simulink model "platoon_greedy_best_first_search"  (R2020b)
settings: Solver=VariableStepAuto  StartTime=0.0  StopTime=25.0  RelTol=1e-3
values from neighbouring files (symbols this model uses):
  loc = zeros(size)    [time_comparison.m]
undefined symbols (not defined in the file or in its folder): objects
libraries: mobileRoboticsLib x13, pid_lib x8
settings Model: Creator=Roozbeh  LastModifiedBy=Roozbeh

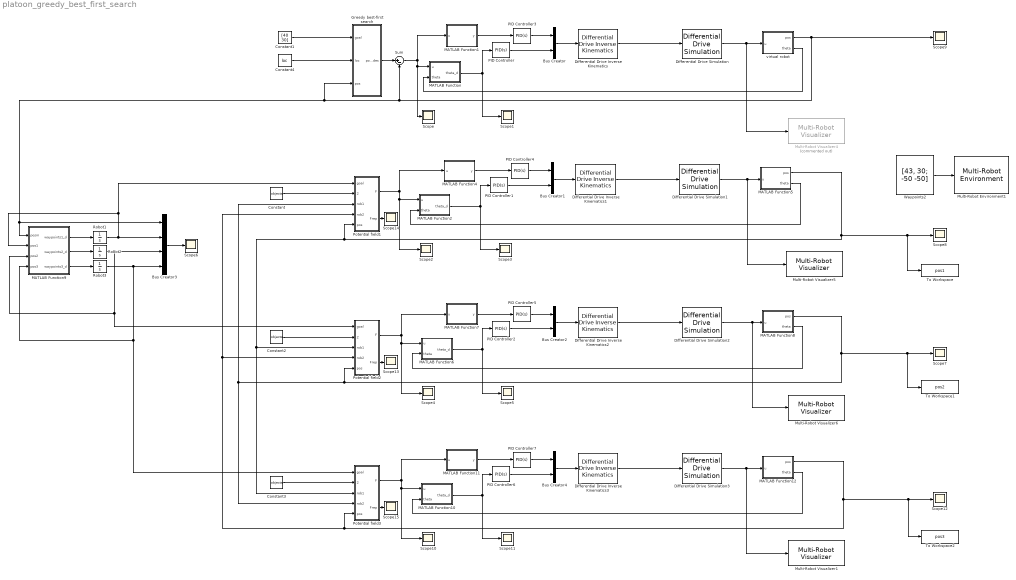
== system platoon_greedy_best_first_search ==
  Bus Creator{,1..2,4} (4 alike) : BusCreator  Inputs=2
  Bus Creator3 : BusCreator  Inputs=4
  Constant : Constant  Value=objects
  Constant1 : Constant  Value=[40 30]
  Constant2 : Constant  Value=objects
  Constant3 : Constant  Value=objects
  Constant4 : Constant  Value=loc
  Differential Drive Inverse Kinematics{,1..3} (4 alike) : mobileRoboticsLib/Kinematic Models/Differential Drive/Differential Drive Inverse Kinematics  wheelRadius=0.1  wheelBase=0.5
      settings: SourceProductName=Mobile Robotics Simulation Toolbox
  Differential Drive Simulation : mobileRoboticsLib/Kinematic Models/Differential Drive/Differential Drive Simulation  wheelRadius=0.1  wheelBase=0.5  initX=6  initY=6  initAngle=0  Ts=0.05
      settings: SourceProductName=Mobile Robotics Simulation Toolbox
  Differential Drive Simulation1 : mobileRoboticsLib/Kinematic Models/Differential Drive/Differential Drive Simulation  wheelRadius=0.1  wheelBase=0.5  initX=8  initY=8  initAngle=0  Ts=0.05
      settings: SourceProductName=Mobile Robotics Simulation Toolbox
  Differential Drive Simulation2 : mobileRoboticsLib/Kinematic Models/Differential Drive/Differential Drive Simulation  wheelRadius=0.1  wheelBase=0.5  initX=4  initY=4  initAngle=0  Ts=0.05
      settings: SourceProductName=Mobile Robotics Simulation Toolbox
  Differential Drive Simulation3 : mobileRoboticsLib/Kinematic Models/Differential Drive/Differential Drive Simulation  wheelRadius=0.1  wheelBase=0.5  initX=4  initY=12  initAngle=0  Ts=0.05
      settings: SourceProductName=Mobile Robotics Simulation Toolbox
  Greedy best-first search : MATLAB Function  TreatAsAtomicUnit=on
  MATLAB Function : MATLAB Function  TreatAsAtomicUnit=on
  MATLAB Function1 : MATLAB Function  TreatAsAtomicUnit=on
  MATLAB Function10 : MATLAB Function  TreatAsAtomicUnit=on
  MATLAB Function11 : MATLAB Function  TreatAsAtomicUnit=on
  MATLAB Function12 : MATLAB Function  TreatAsAtomicUnit=on
  MATLAB Function2 : MATLAB Function  TreatAsAtomicUnit=on
  MATLAB Function4 : MATLAB Function  TreatAsAtomicUnit=on
  MATLAB Function5 : MATLAB Function  TreatAsAtomicUnit=on
  MATLAB Function6 : MATLAB Function  TreatAsAtomicUnit=on
  MATLAB Function7 : MATLAB Function  TreatAsAtomicUnit=on
  MATLAB Function8 : MATLAB Function  TreatAsAtomicUnit=on
  MATLAB Function9 : MATLAB Function  TreatAsAtomicUnit=on
  Multi-Robot Environment1 : mobileRoboticsLib/Environments/Multi-Robot Environment  numRobots=3  mapName=mapRooz  showWaypoints=on  showObjects=off  objectColors=[ 1, 0, 0; 0, 1, 0; 0, 0, 1 ]  objectMarkers='s'  showRobotIds=on  plotSensorLines=on
      settings: SourceProductName=Mobile Robotics Simulation Toolbox
  Multi-Robot Visualizer1 : mobileRoboticsLib/Environments/Multi-Robot Visualizer  idx=3  radius=0.5  robotColor=[0 0 1]  showTraj=off  hasLidar=off  sensorOffset=[0,0]  scanAngles=[-pi/4 0 pi/4]  maxNumScans=0  hasObjDetector=off  objDetectorOffset=[0,0]  objDetectorAngle=0  objDetectorFOV=pi/3  objDetectorMaxRange=5  hasRobotDetector=off  robotDetectorOffset=[0,0]  robotDetectorAngle=0  robotDetectorFOV=pi/3  robotDetectorMaxRange=5  robotDetectorNumDetections=0
      settings: SourceProductName=Mobile Robotics Simulation Toolbox
  Multi-Robot Visualizer4 : mobileRoboticsLib/Environments/Multi-Robot Visualizer  Commented=on  idx=1  radius=0.5  robotColor=[0 0 1]  showTraj=off  hasLidar=off  sensorOffset=[0,0]  scanAngles=[-pi/4 0 pi/4]  maxNumScans=0  hasObjDetector=off  objDetectorOffset=[0,0]  objDetectorAngle=0  objDetectorFOV=pi/3  objDetectorMaxRange=5  hasRobotDetector=off  robotDetectorOffset=[0,0]  robotDetectorAngle=0  robotDetectorFOV=pi/3  robotDetectorMaxRange=5  robotDetectorNumDetections=0
      settings: SourceProductName=Mobile Robotics Simulation Toolbox
  Multi-Robot Visualizer5 : mobileRoboticsLib/Environments/Multi-Robot Visualizer  idx=1  radius=0.5  robotColor=[0 1 0]  showTraj=off  hasLidar=off  sensorOffset=[0,0]  scanAngles=[-pi/4 0 pi/4]  maxNumScans=0  hasObjDetector=off  objDetectorOffset=[0,0]  objDetectorAngle=0  objDetectorFOV=pi/3  objDetectorMaxRange=5  hasRobotDetector=off  robotDetectorOffset=[0,0]  robotDetectorAngle=0  robotDetectorFOV=pi/3  robotDetectorMaxRange=5  robotDetectorNumDetections=0
      settings: SourceProductName=Mobile Robotics Simulation Toolbox
  Multi-Robot Visualizer6 : mobileRoboticsLib/Environments/Multi-Robot Visualizer  idx=2  radius=0.5  robotColor=[1 0 0]  showTraj=off  hasLidar=off  sensorOffset=[0,0]  scanAngles=[-pi/4 0 pi/4]  maxNumScans=0  hasObjDetector=off  objDetectorOffset=[0,0]  objDetectorAngle=0  objDetectorFOV=pi/3  objDetectorMaxRange=5  hasRobotDetector=off  robotDetectorOffset=[0,0]  robotDetectorAngle=0  robotDetectorFOV=pi/3  robotDetectorMaxRange=5  robotDetectorNumDetections=0
      settings: SourceProductName=Mobile Robotics Simulation Toolbox
  PID Controller{,1..2,6} (4 alike) : pid_lib/PID Controller  Controller=PID  Form=Parallel  TimeDomain=Continuous-time  UseExternalTs=off  SampleTime=-1  IntegratorMethod=Forward Euler  FilterMethod=Forward Euler  ControllerParametersSource=internal  P=10  I=1  D=0  UseFilter=on  N=100  TunerSelectOption=Transfer Function Based (PID Tuner App)  InitialConditionSource=internal  InitialConditionForIntegrator=0  InitialConditionForFilter=0  DifferentiatorICPrevScaledInput=0  ExternalReset=none  TrackingMode=off  Kt=1  LimitOutput=off  SatLimitsSource=internal  UpperSaturationLimit=3  LowerSaturationLimit=-3  LinearizeAsGain=on  AntiWindupMode=none  Kb=1  POutMin=[]  POutMax=[]  IOutMin=[]  IOutMax=[]  DOutMin=[]  DOutMax=[]  NOutMin=[]  NOutMax=[]  SumOutMin=[]  SumOutMax=[]  SaturationOutMin=[]  SaturationOutMax=[]  PParamMin=[]  PParamMax=[]  IParamMin=[]  IParamMax=[]  DParamMin=[]  DParamMax=[]  NParamMin=[]  NParamMax=[]  KbParamMin=[]  KbParamMax=[]  KtParamMin=[]  KtParamMax=[]  KbOutMin=[]  KbOutMax=[]  KtOutMin=[]  KtOutMax=[]  IntegratorOutMin=[]  IntegratorOutMax=[]  FilterOutMin=[]  FilterOutMax=[]  SumI1OutMin=[]  SumI1OutMax=[]  SumI2OutMin=[]  SumI2OutMax=[]  SumI3OutMin=[]  SumI3OutMax=[]  SumI4OutMin=[]  SumI4OutMax=[]  SumDOutMin=[]  SumDOutMax=[]  DifferentiatorOutMin=[]  DifferentiatorOutMax=[]  FilterDiffOutCoefMin=[]  FilterDiffOutCoefMax=[]  ReciprocalOutMin=[]  ReciprocalOutMax=[]  SumDenOutMin=[]  SumDenOutMax=[]  SumNumOutMin=[]  SumNumOutMax=[]  DivideOutMin=[]  DivideOutMax=[]  UdiffTsProdOutMin=[]  UdiffTsProdOutMax=[]  NTsProdOutMin=[]  NTsProdOutMax=[]  UintegralTsProdOutMin=[]  UintegralTsProdOutMax=[]  UngainTsProdOutMin=[]  UngainTsProdOutMax=[]  IntegratorContinuousStateAttributes=''  IntegratorStateMustResolveToSignalObject=off  IntegratorRTWStateStorageClass=Auto  FilterContinuousStateAttributes=''  FilterStateMustResolveToSignalObject=off  FilterRTWStateStorageClass=Auto  ParallelPVariant=InternalParameters  IdealPVariant=Disabled  IVariant=InternalParameters  DVariant=InternalParameters  IntegratorVariant=Continuous  SatVariant=Disabled  AWVariant=Passthrough  PCopyVariant=Disabled  TRVariant=Disabled  FdbkBlocksVariant=Forward  IdealPFdbkVariant=Disabled  SatFdbkVariant=Disabled  DerivativeFilterVariant=ContFilter  NVariant=InternalParameters  NCopyVariant=Disabled  FilterICVariant=InternalICsFilter  IntegratorICVariant=InternalICs  ExternalResetVariant=Disabled  TRSumVariant=Passthrough  SumFdbkVariant=Disabled  SumVariant=Sum_PID  TsampFilterVariant=InternalTs  TsampNgainVariant=Passthrough  TsampIntegralVariant=Passthrough  ExternalSaturationOutDataTypeStr=Inherit: Same as second input
  PID Controller3 : pid_lib/PID Controller  Controller=PID  Form=Parallel  TimeDomain=Continuous-time  UseExternalTs=off  SampleTime=-1  IntegratorMethod=Forward Euler  FilterMethod=Forward Euler  ControllerParametersSource=internal  P=5  I=0  D=0.1  UseFilter=on  N=100  TunerSelectOption=Transfer Function Based (PID Tuner App)  InitialConditionSource=internal  InitialConditionForIntegrator=0  InitialConditionForFilter=0  DifferentiatorICPrevScaledInput=0  ExternalReset=none  TrackingMode=off  Kt=1  LimitOutput=on  SatLimitsSource=internal  UpperSaturationLimit=3  LowerSaturationLimit=-3  LinearizeAsGain=on  AntiWindupMode=none  Kb=1  POutMin=[]  POutMax=[]  IOutMin=[]  IOutMax=[]  DOutMin=[]  DOutMax=[]  NOutMin=[]  NOutMax=[]  SumOutMin=[]  SumOutMax=[]  SaturationOutMin=[]  SaturationOutMax=[]  PParamMin=[]  PParamMax=[]  IParamMin=[]  IParamMax=[]  DParamMin=[]  DParamMax=[]  NParamMin=[]  NParamMax=[]  KbParamMin=[]  KbParamMax=[]  KtParamMin=[]  KtParamMax=[]  KbOutMin=[]  KbOutMax=[]  KtOutMin=[]  KtOutMax=[]  IntegratorOutMin=[]  IntegratorOutMax=[]  FilterOutMin=[]  FilterOutMax=[]  SumI1OutMin=[]  SumI1OutMax=[]  SumI2OutMin=[]  SumI2OutMax=[]  SumI3OutMin=[]  SumI3OutMax=[]  SumI4OutMin=[]  SumI4OutMax=[]  SumDOutMin=[]  SumDOutMax=[]  DifferentiatorOutMin=[]  DifferentiatorOutMax=[]  FilterDiffOutCoefMin=[]  FilterDiffOutCoefMax=[]  ReciprocalOutMin=[]  ReciprocalOutMax=[]  SumDenOutMin=[]  SumDenOutMax=[]  SumNumOutMin=[]  SumNumOutMax=[]  DivideOutMin=[]  DivideOutMax=[]  UdiffTsProdOutMin=[]  UdiffTsProdOutMax=[]  NTsProdOutMin=[]  NTsProdOutMax=[]  UintegralTsProdOutMin=[]  UintegralTsProdOutMax=[]  UngainTsProdOutMin=[]  UngainTsProdOutMax=[]  IntegratorContinuousStateAttributes=''  IntegratorStateMustResolveToSignalObject=off  IntegratorRTWStateStorageClass=Auto  FilterContinuousStateAttributes=''  FilterStateMustResolveToSignalObject=off  FilterRTWStateStorageClass=Auto  ParallelPVariant=InternalParameters  IdealPVariant=Disabled  IVariant=InternalParameters  DVariant=InternalParameters  IntegratorVariant=Continuous  SatVariant=Enabled  AWVariant=Passthrough  PCopyVariant=Disabled  TRVariant=Disabled  FdbkBlocksVariant=Forward  IdealPFdbkVariant=Disabled  SatFdbkVariant=Disabled  DerivativeFilterVariant=ContFilter  NVariant=InternalParameters  NCopyVariant=Disabled  FilterICVariant=InternalICsFilter  IntegratorICVariant=InternalICs  ExternalResetVariant=Disabled  TRSumVariant=Passthrough  SumFdbkVariant=Disabled  SumVariant=Sum_PID  TsampFilterVariant=InternalTs  TsampNgainVariant=Passthrough  TsampIntegralVariant=Passthrough  ExternalSaturationOutDataTypeStr=Inherit: Same as second input
  PID Controller4 : pid_lib/PID Controller  Controller=PID  Form=Parallel  TimeDomain=Continuous-time  UseExternalTs=off  SampleTime=-1  IntegratorMethod=Forward Euler  FilterMethod=Forward Euler  ControllerParametersSource=internal  P=5  I=0  D=0.1  UseFilter=on  N=100  TunerSelectOption=Transfer Function Based (PID Tuner App)  InitialConditionSource=internal  InitialConditionForIntegrator=0  InitialConditionForFilter=0  DifferentiatorICPrevScaledInput=0  ExternalReset=none  TrackingMode=off  Kt=1  LimitOutput=on  SatLimitsSource=internal  UpperSaturationLimit=5  LowerSaturationLimit=-5  LinearizeAsGain=on  AntiWindupMode=none  Kb=1  POutMin=[]  POutMax=[]  IOutMin=[]  IOutMax=[]  DOutMin=[]  DOutMax=[]  NOutMin=[]  NOutMax=[]  SumOutMin=[]  SumOutMax=[]  SaturationOutMin=[]  SaturationOutMax=[]  PParamMin=[]  PParamMax=[]  IParamMin=[]  IParamMax=[]  DParamMin=[]  DParamMax=[]  NParamMin=[]  NParamMax=[]  KbParamMin=[]  KbParamMax=[]  KtParamMin=[]  KtParamMax=[]  KbOutMin=[]  KbOutMax=[]  KtOutMin=[]  KtOutMax=[]  IntegratorOutMin=[]  IntegratorOutMax=[]  FilterOutMin=[]  FilterOutMax=[]  SumI1OutMin=[]  SumI1OutMax=[]  SumI2OutMin=[]  SumI2OutMax=[]  SumI3OutMin=[]  SumI3OutMax=[]  SumI4OutMin=[]  SumI4OutMax=[]  SumDOutMin=[]  SumDOutMax=[]  DifferentiatorOutMin=[]  DifferentiatorOutMax=[]  FilterDiffOutCoefMin=[]  FilterDiffOutCoefMax=[]  ReciprocalOutMin=[]  ReciprocalOutMax=[]  SumDenOutMin=[]  SumDenOutMax=[]  SumNumOutMin=[]  SumNumOutMax=[]  DivideOutMin=[]  DivideOutMax=[]  UdiffTsProdOutMin=[]  UdiffTsProdOutMax=[]  NTsProdOutMin=[]  NTsProdOutMax=[]  UintegralTsProdOutMin=[]  UintegralTsProdOutMax=[]  UngainTsProdOutMin=[]  UngainTsProdOutMax=[]  IntegratorContinuousStateAttributes=''  IntegratorStateMustResolveToSignalObject=off  IntegratorRTWStateStorageClass=Auto  FilterContinuousStateAttributes=''  FilterStateMustResolveToSignalObject=off  FilterRTWStateStorageClass=Auto  ParallelPVariant=InternalParameters  IdealPVariant=Disabled  IVariant=InternalParameters  DVariant=InternalParameters  IntegratorVariant=Continuous  SatVariant=Enabled  AWVariant=Passthrough  PCopyVariant=Disabled  TRVariant=Disabled  FdbkBlocksVariant=Forward  IdealPFdbkVariant=Disabled  SatFdbkVariant=Disabled  DerivativeFilterVariant=ContFilter  NVariant=InternalParameters  NCopyVariant=Disabled  FilterICVariant=InternalICsFilter  IntegratorICVariant=InternalICs  ExternalResetVariant=Disabled  TRSumVariant=Passthrough  SumFdbkVariant=Disabled  SumVariant=Sum_PID  TsampFilterVariant=InternalTs  TsampNgainVariant=Passthrough  TsampIntegralVariant=Passthrough  ExternalSaturationOutDataTypeStr=Inherit: Same as second input
  PID Controller5 : pid_lib/PID Controller  Controller=PID  Form=Parallel  TimeDomain=Continuous-time  UseExternalTs=off  SampleTime=-1  IntegratorMethod=Forward Euler  FilterMethod=Forward Euler  ControllerParametersSource=internal  P=5  I=0  D=0.1  UseFilter=on  N=100  TunerSelectOption=Transfer Function Based (PID Tuner App)  InitialConditionSource=internal  InitialConditionForIntegrator=0  InitialConditionForFilter=0  DifferentiatorICPrevScaledInput=0  ExternalReset=none  TrackingMode=off  Kt=1  LimitOutput=on  SatLimitsSource=internal  UpperSaturationLimit=5  LowerSaturationLimit=-5  LinearizeAsGain=on  AntiWindupMode=none  Kb=1  POutMin=[]  POutMax=[]  IOutMin=[]  IOutMax=[]  DOutMin=[]  DOutMax=[]  NOutMin=[]  NOutMax=[]  SumOutMin=[]  SumOutMax=[]  SaturationOutMin=[]  SaturationOutMax=[]  PParamMin=[]  PParamMax=[]  IParamMin=[]  IParamMax=[]  DParamMin=[]  DParamMax=[]  NParamMin=[]  NParamMax=[]  KbParamMin=[]  KbParamMax=[]  KtParamMin=[]  KtParamMax=[]  KbOutMin=[]  KbOutMax=[]  KtOutMin=[]  KtOutMax=[]  IntegratorOutMin=[]  IntegratorOutMax=[]  FilterOutMin=[]  FilterOutMax=[]  SumI1OutMin=[]  SumI1OutMax=[]  SumI2OutMin=[]  SumI2OutMax=[]  SumI3OutMin=[]  SumI3OutMax=[]  SumI4OutMin=[]  SumI4OutMax=[]  SumDOutMin=[]  SumDOutMax=[]  DifferentiatorOutMin=[]  DifferentiatorOutMax=[]  FilterDiffOutCoefMin=[]  FilterDiffOutCoefMax=[]  ReciprocalOutMin=[]  ReciprocalOutMax=[]  SumDenOutMin=[]  SumDenOutMax=[]  SumNumOutMin=[]  SumNumOutMax=[]  DivideOutMin=[]  DivideOutMax=[]  UdiffTsProdOutMin=[]  UdiffTsProdOutMax=[]  NTsProdOutMin=[]  NTsProdOutMax=[]  UintegralTsProdOutMin=[]  UintegralTsProdOutMax=[]  UngainTsProdOutMin=[]  UngainTsProdOutMax=[]  IntegratorContinuousStateAttributes=''  IntegratorStateMustResolveToSignalObject=off  IntegratorRTWStateStorageClass=Auto  FilterContinuousStateAttributes=''  FilterStateMustResolveToSignalObject=off  FilterRTWStateStorageClass=Auto  ParallelPVariant=InternalParameters  IdealPVariant=Disabled  IVariant=InternalParameters  DVariant=InternalParameters  IntegratorVariant=Continuous  SatVariant=Enabled  AWVariant=Passthrough  PCopyVariant=Disabled  TRVariant=Disabled  FdbkBlocksVariant=Forward  IdealPFdbkVariant=Disabled  SatFdbkVariant=Disabled  DerivativeFilterVariant=ContFilter  NVariant=InternalParameters  NCopyVariant=Disabled  FilterICVariant=InternalICsFilter  IntegratorICVariant=InternalICs  ExternalResetVariant=Disabled  TRSumVariant=Passthrough  SumFdbkVariant=Disabled  SumVariant=Sum_PID  TsampFilterVariant=InternalTs  TsampNgainVariant=Passthrough  TsampIntegralVariant=Passthrough  ExternalSaturationOutDataTypeStr=Inherit: Same as second input
  PID Controller7 : pid_lib/PID Controller  Controller=PID  Form=Parallel  TimeDomain=Continuous-time  UseExternalTs=off  SampleTime=-1  IntegratorMethod=Forward Euler  FilterMethod=Forward Euler  ControllerParametersSource=internal  P=5  I=0  D=0.1  UseFilter=on  N=100  TunerSelectOption=Transfer Function Based (PID Tuner App)  InitialConditionSource=internal  InitialConditionForIntegrator=0  InitialConditionForFilter=0  DifferentiatorICPrevScaledInput=0  ExternalReset=none  TrackingMode=off  Kt=1  LimitOutput=on  SatLimitsSource=internal  UpperSaturationLimit=5  LowerSaturationLimit=-5  LinearizeAsGain=on  AntiWindupMode=none  Kb=1  POutMin=[]  POutMax=[]  IOutMin=[]  IOutMax=[]  DOutMin=[]  DOutMax=[]  NOutMin=[]  NOutMax=[]  SumOutMin=[]  SumOutMax=[]  SaturationOutMin=[]  SaturationOutMax=[]  PParamMin=[]  PParamMax=[]  IParamMin=[]  IParamMax=[]  DParamMin=[]  DParamMax=[]  NParamMin=[]  NParamMax=[]  KbParamMin=[]  KbParamMax=[]  KtParamMin=[]  KtParamMax=[]  KbOutMin=[]  KbOutMax=[]  KtOutMin=[]  KtOutMax=[]  IntegratorOutMin=[]  IntegratorOutMax=[]  FilterOutMin=[]  FilterOutMax=[]  SumI1OutMin=[]  SumI1OutMax=[]  SumI2OutMin=[]  SumI2OutMax=[]  SumI3OutMin=[]  SumI3OutMax=[]  SumI4OutMin=[]  SumI4OutMax=[]  SumDOutMin=[]  SumDOutMax=[]  DifferentiatorOutMin=[]  DifferentiatorOutMax=[]  FilterDiffOutCoefMin=[]  FilterDiffOutCoefMax=[]  ReciprocalOutMin=[]  ReciprocalOutMax=[]  SumDenOutMin=[]  SumDenOutMax=[]  SumNumOutMin=[]  SumNumOutMax=[]  DivideOutMin=[]  DivideOutMax=[]  UdiffTsProdOutMin=[]  UdiffTsProdOutMax=[]  NTsProdOutMin=[]  NTsProdOutMax=[]  UintegralTsProdOutMin=[]  UintegralTsProdOutMax=[]  UngainTsProdOutMin=[]  UngainTsProdOutMax=[]  IntegratorContinuousStateAttributes=''  IntegratorStateMustResolveToSignalObject=off  IntegratorRTWStateStorageClass=Auto  FilterContinuousStateAttributes=''  FilterStateMustResolveToSignalObject=off  FilterRTWStateStorageClass=Auto  ParallelPVariant=InternalParameters  IdealPVariant=Disabled  IVariant=InternalParameters  DVariant=InternalParameters  IntegratorVariant=Continuous  SatVariant=Enabled  AWVariant=Passthrough  PCopyVariant=Disabled  TRVariant=Disabled  FdbkBlocksVariant=Forward  IdealPFdbkVariant=Disabled  SatFdbkVariant=Disabled  DerivativeFilterVariant=ContFilter  NVariant=InternalParameters  NCopyVariant=Disabled  FilterICVariant=InternalICsFilter  IntegratorICVariant=InternalICs  ExternalResetVariant=Disabled  TRSumVariant=Passthrough  SumFdbkVariant=Disabled  SumVariant=Sum_PID  TsampFilterVariant=InternalTs  TsampNgainVariant=Passthrough  TsampIntegralVariant=Passthrough  ExternalSaturationOutDataTypeStr=Inherit: Same as second input
  Potential field1 : MATLAB Function  TreatAsAtomicUnit=on
  Potential field2 : MATLAB Function  TreatAsAtomicUnit=on
  Potential field3 : MATLAB Function  TreatAsAtomicUnit=on
  Robot1 : Integrator  InitialCondition=[8 8]
  Robot2 : Integrator  InitialCondition=[4 5]
  Robot3 : Integrator  InitialCondition=[4 11]
  Scope{,1..15} (16 alike) : Scope
  Sum : Sum  Inputs=|+-
  To Workspace : ToWorkspace  VariableName=pos1  SaveFormat=Timeseries  SampleTime=-1
  To Workspace1 : ToWorkspace  VariableName=pos2  SaveFormat=Timeseries  SampleTime=-1
  To Workspace2 : ToWorkspace  VariableName=pos3  SaveFormat=Timeseries  SampleTime=-1
  Waypoints2 : Constant  Value=[43, 30; -50 -50]
  virtual robot : MATLAB Function  TreatAsAtomicUnit=on
  wires:
  Greedy best-first search/1(pos_des) -> Sum/1
  Sum/1 -> Scope/1, MATLAB Function/1(u), MATLAB Function1/1(u)
  Constant4/1 -> Greedy best-first search/2(loc)
  MATLAB Function12/1(pos) -> To Workspace2/1, Scope12/1, Potential field1/4(rob2), Potential field2/4(rob2), Potential field3/5(pos)
  Waypoints2/1 -> Multi-Robot Environment1/1
  Potential field2/1(F) -> Scope4/1, MATLAB Function6/1(u), MATLAB Function7/1(u)
  Differential Drive Inverse Kinematics3/1 -> Differential Drive Simulation3/1
  Bus Creator4/1 -> Differential Drive Inverse Kinematics3/1
  MATLAB Function5/2(theta) -> MATLAB Function2/2(theta)
  PID Controller5/1 -> Bus Creator2/1
  PID Controller7/1 -> Bus Creator4/1
  MATLAB Function7/1(y) -> PID Controller5/1
  Robot2/1 -> MATLAB Function9/3(pos2), Potential field2/1(goal), Bus Creator3/3
  Constant/1 -> Potential field1/2(objects)
  Differential Drive Simulation3/1 -> Multi-Robot Visualizer1/1, MATLAB Function12/1(u)
  PID Controller/1 -> Bus Creator/2
  MATLAB Function10/1(theta_d) -> PID Controller6/1, Scope11/1
  Differential Drive Simulation1/1 -> Multi-Robot Visualizer5/1, MATLAB Function5/1(u)
  Potential field2/2(Frep) -> Scope13/1
  MATLAB Function6/1(theta_d) -> PID Controller2/1, Scope5/1
  MATLAB Function5/1(pos) -> To Workspace/1, Scope8/1, Potential field1/5(pos), Potential field3/3(rob1), Potential field2/3(rob1)
  MATLAB Function9/1(waypoints1_d) -> Robot1/1
  Constant2/1 -> Potential field2/2(objects)
  PID Controller1/1 -> Bus Creator1/2
  MATLAB Function/1(theta_d) -> PID Controller/1, Scope1/1
  Differential Drive Inverse Kinematics1/1 -> Differential Drive Simulation1/1
  Constant3/1 -> Potential field3/2(objects)
  MATLAB Function1/1(y) -> PID Controller3/1
  PID Controller6/1 -> Bus Creator4/2
  Differential Drive Simulation2/1 -> Multi-Robot Visualizer6/1, MATLAB Function8/1(u)
  Potential field3/1(F) -> Scope10/1, MATLAB Function10/1(u), MATLAB Function11/1(u)
  MATLAB Function11/1(y) -> PID Controller7/1
  Differential Drive Inverse Kinematics/1 -> Differential Drive Simulation/1
  MATLAB Function4/1(y) -> PID Controller4/1
  Differential Drive Inverse Kinematics2/1 -> Differential Drive Simulation2/1
  Bus Creator1/1 -> Differential Drive Inverse Kinematics1/1
  Bus Creator/1 -> Differential Drive Inverse Kinematics/1
  Potential field1/1(F) -> Scope2/1, MATLAB Function2/1(u), MATLAB Function4/1(u)
  Robot3/1 -> MATLAB Function9/4(pos3), Potential field3/1(goal), Bus Creator3/4
  MATLAB Function2/1(theta_d) -> PID Controller1/1, Scope3/1
  Bus Creator2/1 -> Differential Drive Inverse Kinematics2/1
  MATLAB Function12/2(theta) -> MATLAB Function10/2(theta)
  Potential field3/2(Frep) -> Scope15/1
  MATLAB Function9/2(waypoints2_d) -> Robot2/1
  PID Controller2/1 -> Bus Creator2/2
  Differential Drive Simulation/1 -> Multi-Robot Visualizer4/1, virtual robot/1(u)
  virtual robot/1(pos) -> Greedy best-first search/3(pos), MATLAB Function9/1(posm), Bus Creator3/1, Sum/2, Scope9/1
  Potential field1/2(Frep) -> Scope14/1
  PID Controller3/1 -> Bus Creator/1
  Robot1/1 -> Potential field1/1(goal), MATLAB Function9/2(pos1), Bus Creator3/2
  virtual robot/2(theta) -> MATLAB Function/2(theta)
  Bus Creator3/1 -> Scope6/1
  MATLAB Function9/3(waypoints3_d) -> Robot3/1
  PID Controller4/1 -> Bus Creator1/1
  MATLAB Function8/2(theta) -> MATLAB Function6/2(theta)
  MATLAB Function8/1(pos) -> To Workspace1/1, Scope7/1, Potential field1/3(rob1), Potential field3/4(rob2), Potential field2/5(pos)
  Constant1/1 -> Greedy best-first search/1(goal)

== matlab function platoon_greedy_best_first_search/MATLAB Function10 ==
  data: u input; theta_d output; theta input
function theta_d = fcn(u, theta)

delta = atan2(u(2), u(1)) - theta;
sgn = sign(delta);
delta_hat = delta - 2*pi*sgn;
if abs(delta_hat) < abs(delta)
    theta_d = delta_hat;
else
    theta_d = delta;
end

== matlab function platoon_greedy_best_first_search/MATLAB Function11 ==
  data: u input; y output
function y = fcn(u)

y = sqrt(u(1)^2 + u(2)^2);

== matlab function platoon_greedy_best_first_search/MATLAB Function12 ==
  data: u input; pos output; theta output
function [pos, theta] = fcn(u)

pos = u(1:2);
theta = u(3);

== matlab function platoon_greedy_best_first_search/Potential field1 ==
  data: goal input; objects input; rob1 input; rob2 input; pos input; F output; Frep output
function [F, Frep]  = fcn(goal, objects, rob1, rob2, pos)
% initialization - user variables
zeta = 1;
d = 3;
etha = 20;
ro = 4;

objects = [objects; rob1'; rob2'];

% att
dist = pos - goal;
dist_norm = norm(dist);
if dist_norm > d
    Fatt = -d*zeta*dist/dist_norm;
else
    Fatt = -zeta*dist;
end

% repel
Frep = [0; 0];
for i = 1:1:size(objects,1)
    dist_obj = objects(i,:)' - pos;
    dist_obj_norm = norm(dist_obj);
    if dist_obj_norm < ro
        Frep = Frep + etha*(1/dist_obj_norm - 1/ro) * dist_obj / (dist_obj_norm^3);
    end
end

% total
F = Fatt - Frep;

== matlab function platoon_greedy_best_first_search/Potential field2 ==
  data: goal input; objects input; rob1 input; rob2 input; pos input; F output; Frep output
function [F, Frep]  = fcn(goal, objects, rob1, rob2, pos)
% initialization - user variables
zeta = 1;
d = 3;
etha = 20;
ro = 4;

objects = [objects; rob1'; rob2'];

% att
dist = pos - goal;
dist_norm = norm(dist);
if dist_norm > d
    Fatt = -d*zeta*dist/dist_norm;
else
    Fatt = -zeta*dist;
end

% repel
Frep = [0; 0];
for i = 1:1:size(objects,1)
    dist_obj = objects(i,:)' - pos;
    dist_obj_norm = norm(dist_obj);
    if dist_obj_norm < ro
        Frep = Frep + etha*(1/dist_obj_norm - 1/ro) * dist_obj / (dist_obj_norm^3);
    end
end

% total
F = Fatt - Frep;

== matlab function platoon_greedy_best_first_search/Potential field3 ==
  data: goal input; objects input; rob1 input; rob2 input; pos input; F output; Frep output
function [F, Frep]  = fcn(goal, objects, rob1, rob2, pos)
% initialization - user variables
zeta = 1;
d = 3;
etha = 20;
ro = 4;

objects = [objects; rob1'; rob2'];

% att
dist = pos - goal;
dist_norm = norm(dist);
if dist_norm > d
    Fatt = -d*zeta*dist/dist_norm;
else
    Fatt = -zeta*dist;
end

% repel
Frep = [0; 0];
for i = 1:1:size(objects,1)
    dist_obj = objects(i,:)' - pos;
    dist_obj_norm = norm(dist_obj);
    
    if dist_obj_norm < ro
        Frep = Frep + etha*(1/dist_obj_norm - 1/ro) * dist_obj / (dist_obj_norm^3);
    end
end

% total
F = Fatt - Frep;

== matlab function platoon_greedy_best_first_search/MATLAB Function ==
  data: u input; theta_d output; theta input
function theta_d = fcn(u, theta)

delta = atan2(u(2), u(1)) - theta;
sgn = sign(delta);
delta_hat = delta - 2*pi*sgn;
if abs(delta_hat) < abs(delta)
    theta_d = delta_hat;
else
    theta_d = delta;
end

== matlab function platoon_greedy_best_first_search/Greedy best-first search ==
  data: goal input; loc input; pos input; pos_des output
function pos_des = Greedy_best_first_search(goal, loc, pos)
% f(s) = h(s)
% h(s): estimated cost of the cheapest path from s to goal_state => 
% h(s) = norm(pos(s) - pos(goal))
% Actions = {N, S, E, W, NW, NE, SW, SE} |A| = 8
actions = [0 1; 0 -1; 1 0; -1 0; -1 1; 1 1; -1 -1; 1 -1]; % direction of Actions in x-y coordination
numActions = size(actions,1);
m = size(loc,1);
n = size(loc,2);
goal_state = round(goal');
start_state = round(pos');
s = start_state;
parent = zeros(m, n);
f = ones(m, n)*m*n;
visited = zeros(m, n);

while ~(s(1) == goal_state(1) && s(2) == goal_state(2))
    visited(s(1), s(2)) = 1;
    f(s(1), s(2)) = m*n;
    % updating nodes
    for a = 1:numActions
        sp = s + actions(a,:);
        if sp(1) < 1 || sp(1) > size(loc,1) || sp(2) < 1 || sp(2) > size(loc,2) ...
                || visited(sp(1), sp(2)) == 1 || loc(sp(1), sp(2)) == 1
            continue
        end
        h = norm(goal_state - sp);
        if h < f(sp(1), sp(2))
            f(sp(1), sp(2)) = h;
            parent(sp(1), sp(2)) = (s(2)-1)*m + s(1);
        end
    end
    % searching
    M = min(f,[], 'all');
    [x, y] = find(f==M);
    s = [x(1) y(1)];
%     fprintf('s = (%d, %d): f = %d)\n', s(1), s(2), M);
end

% constructing path
path = zeros(m*n, 2);
path(m*n,:) = s;
i = m*n;
while ~(s(1) == start_state(1) && s(2) == start_state(2))
    sp = parent(s(1), s(2));
    s = [mod(sp,m) ceil(sp/m)];
    i = i - 1;
    path(i,:) = s;
    %fprintf('s = (%d, %d)\n', s(1), s(2))
end

[x, ~] = find(path==0);
path = path(x(size(x,1)) + 1:m*n,:);
if size(path,1) == 1
    pos_des = path(1,:);
else
    pos_des = path(2,:);
end


end

== matlab function platoon_greedy_best_first_search/MATLAB Function1 ==
  data: u input; y output
function y = fcn(u)

y = 0.5*sqrt(u(1)^2 + u(2)^2);

== matlab function platoon_greedy_best_first_search/virtual robot ==
  data: u input; pos output; theta output
function [pos, theta] = fcn(u)

pos = u(1:2);
theta = u(3);

== matlab function platoon_greedy_best_first_search/MATLAB Function2 ==
  data: u input; theta_d output; theta input
function theta_d = fcn(u, theta)

delta = atan2(u(2), u(1)) - theta;
sgn = sign(delta);
delta_hat = delta - 2*pi*sgn;
if abs(delta_hat) < abs(delta)
    theta_d = delta_hat;
else
    theta_d = delta;
end

== matlab function platoon_greedy_best_first_search/MATLAB Function4 ==
  data: u input; y output
function y = fcn(u)

y = sqrt(u(1)^2 + u(2)^2);

== matlab function platoon_greedy_best_first_search/MATLAB Function5 ==
  data: u input; pos output; theta output
function [pos, theta] = fcn(u)

pos = u(1:2);
theta = u(3);

== matlab function platoon_greedy_best_first_search/MATLAB Function6 ==
  data: u input; theta_d output; theta input
function theta_d = fcn(u, theta)

delta = atan2(u(2), u(1)) - theta;
sgn = sign(delta);
delta_hat = delta - 2*pi*sgn;
if abs(delta_hat) < abs(delta)
    theta_d = delta_hat;
else
    theta_d = delta;
end

== matlab function platoon_greedy_best_first_search/MATLAB Function7 ==
  data: u input; y output
function y = fcn(u)

y = sqrt(u(1)^2 + u(2)^2);

== matlab function platoon_greedy_best_first_search/MATLAB Function8 ==
  data: u input; pos output; theta output
function [pos, theta] = fcn(u)

pos = u(1:2);
theta = u(3);

== matlab function platoon_greedy_best_first_search/MATLAB Function9 ==
  data: posm input; waypoints1_d output; pos1 input; waypoints2_d output; pos2 input; pos3 input; waypoints3_d output
function [waypoints1_d, waypoints2_d, waypoints3_d] = fcn(posm, pos1, pos2, pos3)

L = [-3 1 1 1; 1 -3 1 1; 1 1 -3 1; 1 1 1 -3];
F = [-3 0; 0 0; -4 -3; -4 3];
x = [posm(1:2)'; pos1(1:2)'; pos2(1:2)'; pos3(1:2)'];
xd = L*(x - F);

waypoints1_d = xd(2,:);
waypoints2_d = xd(3,:);
waypoints3_d = xd(4,:);
